simulink model "LqrTenzoWMotors"  (R2017a)
settings: Solver=ode23  StartTime=0.0  StopTime=15  RelTol=1e-3  EnableMultiTasking=on
values from neighbouring files (symbols this model uses):
  A0 = tenzo_min_nominale.a    [HTenzoV10.m]    (also in HTenzoV11.m; HTenzoV12.m; HTenzoV13.m; HTenzoV14.m)
  amplitudeNoise = 2    [HTenzoV10.m]    (also in HTenzoV11.m; HTenzoV12.m; HTenzoV13.m; HTenzoV14.m)
  amplitudePertIN = 0    [HTenzoV10.m]    (also in HTenzoV11.m; HTenzoV12.m; HTenzoV13.m; HTenzoV14.m)
  amplitudePertOut = 0    [HTenzoV10.m]    (also in HTenzoV11.m; HTenzoV12.m; HTenzoV13.m; HTenzoV14.m)
  Aoss = tenzo_min_nominale.a-L_3*tenzo_min_nominale.c    [HTenzoV10.m]    (also in HTenzoV11.m; HTenzoV12.m = tenzo_min_nominale.a-V*tenzo_min_nominale.c; HTenzoV13.m = tenzo_min_nominale.a-V*tenzo_min_nominale.c; HTenzoV14.m = tenzo_min_nominale.a-V*tenzo_min_nominale.c)
  B0 = tenzo_min_nominale.b    [HTenzoV10.m]    (also in HTenzoV11.m; HTenzoV12.m; HTenzoV13.m; HTenzoV14.m)
  Bossw = [tenzo_min_nominale.b-L_3*D L_3]    [HTenzoV10.m]    (also in HTenzoV11.m; HTenzoV12.m = [tenzo_min_nominale.b-V*D V]; HTenzoV13.m = [tenzo_min_nominale.b-V*D V]; HTenzoV14.m = [tenzo_min_nominale.b-V*D V])
  C0 = tenzo_min_nominale.c    [HTenzoV10.m]    (also in HTenzoV11.m; HTenzoV12.m; HTenzoV13.m; HTenzoV14.m)
  Coss = eye(size(Aoss,1))    [HTenzoV10.m]    (also in HTenzoV11.m; HTenzoV12.m; HTenzoV13.m; HTenzoV14.m)
  cstPertIn = 0    [HTenzoV10.m]    (also in HTenzoV11.m; HTenzoV12.m; HTenzoV13.m; HTenzoV14.m)
  cstPertOut = 0    [HTenzoV10.m]    (also in HTenzoV11.m; HTenzoV12.m; HTenzoV13.m; HTenzoV14.m)
  D0 = tenzo_min_nominale.d    [HTenzoV10.m]    (also in HTenzoV11.m; HTenzoV12.m; HTenzoV13.m; HTenzoV14.m)
  Doss = zeros(size(Aoss,1),poss)    [HTenzoV10.m]    (also in HTenzoV11.m; HTenzoV12.m; HTenzoV13.m; HTenzoV14.m)
  Kopt = Kopt_3    [HTenzoV10.m]    (also in HTenzoV11.m; HTenzoV12.m; HTenzoV13.m; HTenzoV14.m)
  omegaPertIN = 6    [HTenzoV10.m]    (also in HTenzoV11.m; HTenzoV12.m; HTenzoV13.m; HTenzoV14.m)
  omegaPertOut = 0.1    [HTenzoV10.m]    (also in HTenzoV11.m; HTenzoV12.m; HTenzoV13.m; HTenzoV14.m)
undefined symbols (not defined in the file or in its folder): sigbuilder_block
settings Model: SimulationMode=accelerator  Creator=danilo  LastModifiedBy=userk
settings DataIOCC: LimitDataPoints=on  SaveFormat=Array
settings OptimizationCC: ExpressionDepthLimit=2147483647  LifeSpan=inf
settings DebuggingCC: UnderspecifiedInitializationDetection=Classic  MergeDetectMultiDrivingBlocksExec=none  SolverPrmCheckMsg=warning  FcnCallInpInsideContextMsg=warning  AllowSymbolicDim=off  StateNameClashWarn=warning  SFUnexpectedBacktrackingDiag=warning  SFNoUnconditionalDefaultTransitionDiag=warning  SFExecutionAtInitializationDiag=none
settings HardwareCC: ProdBitPerPointer=32  ProdBitPerSizeT=32  ProdBitPerPtrDiffT=32  ProdLargestAtomicFloat=None  ProdIntDivRoundTo=Undefined  ProdEndianess=Unspecified  ProdWordSize=32  ProdHWDeviceType=32-bit Generic
settings ModelReferenceCC: PropagateSignalLabelsOutOfModel=off
settings GRTTargetCC: TargetLangStandard=C89/C90 (ANSI)  GeneratePreprocessorConditionals=Disable all  CombineOutputUpdateFcns=off  GRTInterface=on
settings ConfigComp: CovMetricSettings=dw  CovHtmlReporting=on  CovSaveCumulativeToWorkspaceVar=on  CovSaveSingleToWorkspaceVar=on  CovExternalEMLEnable=off

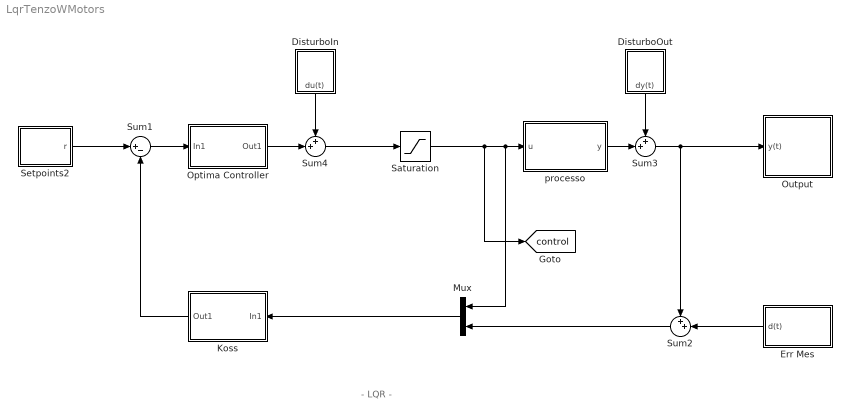
== system LqrTenzoWMotors ==
  note: - LQR -
  DisturboIn : Subsystem
  DisturboOut : Subsystem
  Err Mes : Subsystem
  Koss : Subsystem
  Mux : Mux  Inputs=2
  Optima Controller : Subsystem
  Output : Subsystem
  Saturation : Saturate  UpperLimit=36000000  LowerLimit=-36000000
  Setpoints2 : Subsystem
  Sum1 : Sum  Inputs=|+-
  Sum2 : Sum  Inputs=++|
  Sum3 : Sum  Inputs=++|
  Sum4 : Sum  Inputs=++|
  processo : Subsystem
  tag scope: control=global
  wires:
  Setpoints2/1(r) -> Sum1/1
  Err Mes/1("  d(t)") -> Sum2/2
  Sum2/1 -> Mux/2
  processo/1(y) -> Sum3/2
  Sum3/1 -> Sum2/1, Output/1(y(t))
  DisturboOut/1("dy(t) ") -> Sum3/1
  Sum1/1 -> Optima Controller/1(In1)
  Optima Controller/1(Out1) -> Sum4/2
  Mux/1 -> Koss/1(In1)
  Koss/1(Out1) -> Sum1/2
  DisturboIn/1(du(t)) -> Sum4/1
  Sum4/1 -> Saturation/1
  Saturation/1 -> [control], Mux/1, processo/1(u)

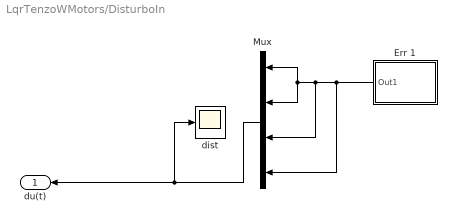
== system LqrTenzoWMotors/DisturboIn ==
  Err 1 : Subsystem
  Mux : Mux  Inputs=[1 1 1 1]
  dist : Scope
  du(t) : Outport
  wires:
  Mux/1 -> dist/1, du(t)/1
  Err 1/1(Out1) -> Mux/4, Mux/3, Mux/2, Mux/1

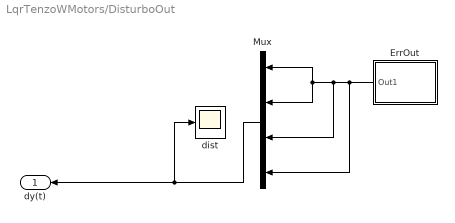
== system LqrTenzoWMotors/DisturboOut ==
  ErrOut : Subsystem
  Mux : Mux  Inputs=[1 1 1 1]
  dist : Scope
  "dy(t) " : Outport
  wires:
  ErrOut/1(Out1) -> Mux/4, Mux/3, Mux/2, Mux/1
  Mux/1 -> "dy(t) "/1, dist/1

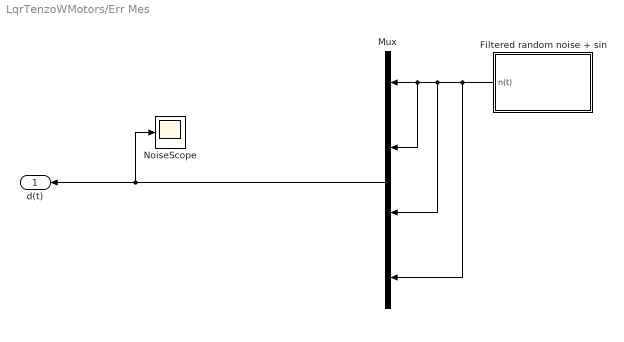
== system LqrTenzoWMotors/Err Mes ==
  Filtered random noise + sin : Subsystem
  Mux : Mux  Inputs=[1 1 1 1]
  NoiseScope : Scope
  "  d(t)" : Outport
  wires:
  Mux/1 -> NoiseScope/1, "  d(t)"/1
  Filtered random noise + sin/1(n(t)) -> Mux/4, Mux/3, Mux/2, Mux/1

== system LqrTenzoWMotors/Koss ==
  In1 : Inport
  "abc " : StateSpace  A=Aoss  B=Bossw  C=Coss  D=Doss  X0=0
  Out1 : Outport
  wires:
  In1/1 -> "abc "/1
  "abc "/1 -> Out1/1

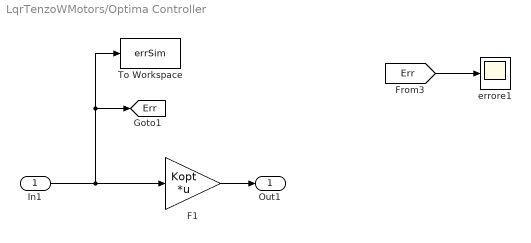
== system LqrTenzoWMotors/Optima Controller ==
  In1 : Inport
  F1 : Gain  Gain=Kopt  Multiplication=Matrix(K*u) (u vector)
  To Workspace : ToWorkspace  VariableName=errSim  SaveFormat=Structure  SampleTime=-1
  errore1 : Scope
  Out1 : Outport
  tag scope: Err=global
  wires:
  In1/1 -> F1/1, To Workspace/1, [Err]
  F1/1 -> Out1/1
  [Err] -> errore1/1

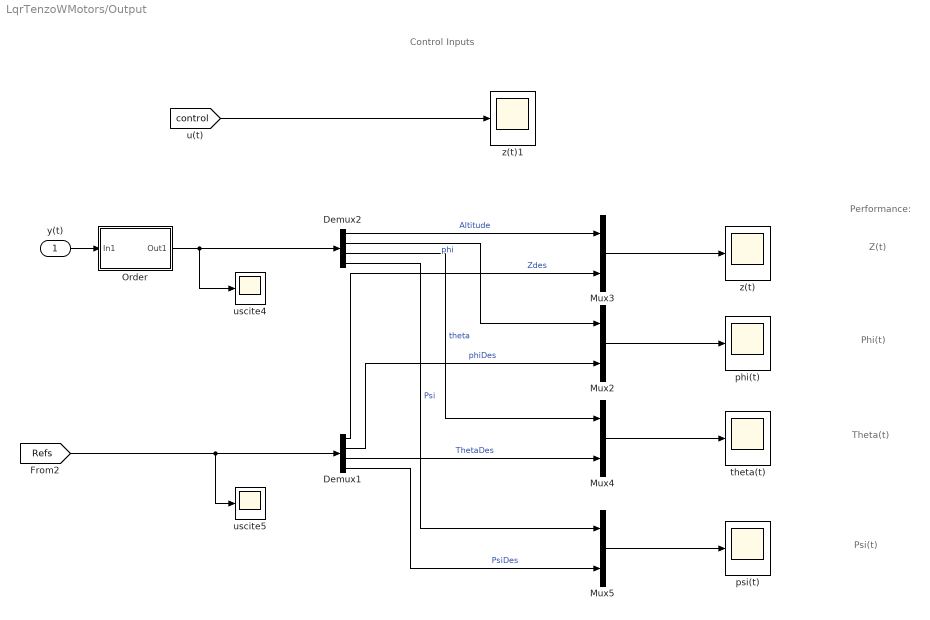
== system LqrTenzoWMotors/Output ==
  note: Psi(t)
  note: Theta(t)
  note: Phi(t)
  note: Performance:
  note: Z(t)
  note: Control Inputs
  y(t) : Inport
  Demux1 : Demux
  Demux2 : Demux
  Mux{2..5} (4 alike) : Mux  Inputs=2
  "Order " : Subsystem
  phi(t) : Scope
  psi(t) : Scope
  theta(t) : Scope
  uscite4 : Scope
  uscite5 : Scope
  z(t) : Scope
  z(t)1 : Scope
  wires:
  [Refs] -> Demux1/1, uscite5/1
  Demux1/1 -> Mux3/2  "Zdes"
  Mux2/1 -> phi(t)/1
  Demux2/2 -> Mux2/1  "phi"
  Mux3/1 -> z(t)/1
  Demux2/1 -> Mux3/1  "Altitude"
  Mux4/1 -> theta(t)/1
  Demux2/3 -> Mux4/1  "theta"
  Mux5/1 -> psi(t)/1
  Demux2/4 -> Mux5/1  "Psi"
  Demux1/2 -> Mux2/2  "phiDes"
  Demux1/3 -> Mux4/2  "ThetaDes"
  Demux1/4 -> Mux5/2  "PsiDes"
  "Order "/1(Out1) -> Demux2/1, uscite4/1
  y(t)/1 -> "Order "/1(In1)
  [control] -> z(t)1/1

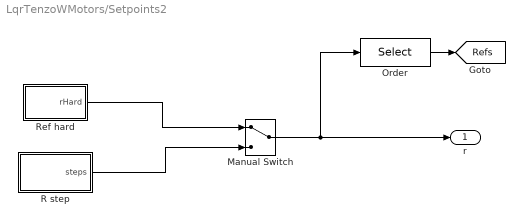
== system LqrTenzoWMotors/Setpoints2 ==
  Manual Switch : ManualSwitch
  Order : Selector  InputPortWidth=8  IndexOptions=Index vector (dialog)  Indices=[1,3,4,5]  OutputSizes=1
  R step : Subsystem
  "Ref hard " : Subsystem
  r : Outport
  tag scope: Refs=global
  wires:
  "Ref hard "/1(rHard) -> Manual Switch/1
  R step/1("steps ") -> Manual Switch/2
  Manual Switch/1 -> Order/1, r/1
  Order/1 -> [Refs]

== system LqrTenzoWMotors/processo ==
  u : Inport
  Processo1 : StateSpace  A=A0  B=B0  C=C0  D=D0  X0=0
  "u(t) " : Scope
  y : Outport
  wires:
  u/1 -> "u(t) "/1, Processo1/1
  Processo1/1 -> y/1

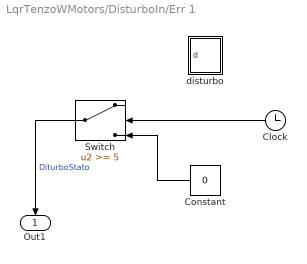
== system LqrTenzoWMotors/DisturboIn/Err 1 ==
  Clock : Clock
  Constant : Constant  Value=0
  Switch : Switch  Threshold=5
  disturbo : Subsystem
  Out1 : Outport
  wires:
  Constant/1 -> Switch/3
  Switch/1 -> Out1/1  "DiturboStato"
  Clock/1 -> Switch/2

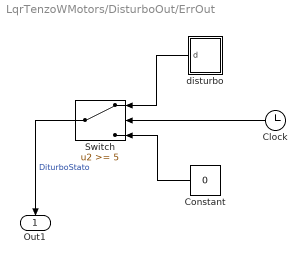
== system LqrTenzoWMotors/DisturboOut/ErrOut ==
  Clock : Clock
  Constant : Constant  Value=0
  Switch : Switch  Threshold=5
  disturbo : Subsystem
  Out1 : Outport
  wires:
  Clock/1 -> Switch/2
  Switch/1 -> Out1/1  "DiturboStato"
  disturbo/1(d) -> Switch/1
  Constant/1 -> Switch/3

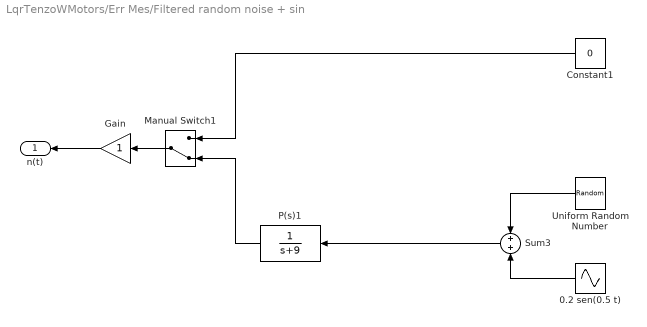
== system LqrTenzoWMotors/Err Mes/Filtered random noise + sin ==
  0.2 sen(0.5 t) : Sin  Amplitude=amplitudeNoise  Frequency=65  Phase=1  SampleTime=0
  Constant1 : Constant  Value=0
  Gain : Gain
  Manual Switch1 : ManualSwitch  CurrentSetting=0
  P(s)1 : TransferFcn  Numerator=1  Denominator=[1 9]
  Sum3 : Sum
  Uniform Random Number : UniformRandomNumber  Minimum=-10  Maximum=10  SampleTime=0.1
  n(t) : Outport
  wires:
  Uniform Random Number/1 -> Sum3/1
  Constant1/1 -> Manual Switch1/1
  Sum3/1 -> P(s)1/1
  Gain/1 -> n(t)/1
  P(s)1/1 -> Manual Switch1/2
  Manual Switch1/1 -> Gain/1
  0.2 sen(0.5 t)/1 -> Sum3/2

== system LqrTenzoWMotors/Output/Order  ==
  In1 : Inport
  Demux3 : Demux
  Mux1 : Mux
  Out1 : Outport
  wires:
  Demux3/2 -> Mux1/3
  Demux3/1 -> Mux1/2
  In1/1 -> Demux3/1
  Mux1/1 -> Out1/1
  Demux3/4 -> Mux1/1
  Demux3/3 -> Mux1/4

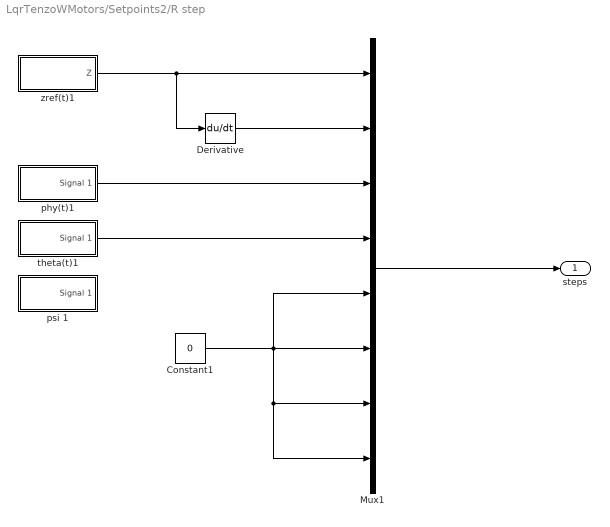
== system LqrTenzoWMotors/Setpoints2/R step ==
  Constant1 : Constant  Value=0
  Derivative : Derivative
  Mux1 : Mux  Inputs=[1 1 1 1 1 1 1 1]
  phy(t)1 : Subsystem  Tag=STV Subsys  LoadFcn=sigbuilder_block('load');  StartFcn=sigbuilder_block('start');  StopFcn=sigbuilder_block('stop');  ClipboardFcn=sigbuilder_block('clipboard');  mask(Sigbuilder block){tuvar=[0:10]}
      mask help: Simulink:masks:SigbuilderBlock_MD
      mask init:
      | if ~strcmp(get_param(bdroot(gcbh),'SimulationStatus'),'stopped') tuvar = sigbuilder_block('maskInit'); end
      settings: CopyFcn=sigbuilder_block('copy');  DeleteFcn=sigbuilder_block('delete');  ModelCloseFcn=sigbuilder_block('modelClose');  PreSaveFcn=sigbuilder_block('preSave');  PauseFcn=sigbuilder_block('pause');  ContinueFcn=sigbuilder_block('continue');  NameChangeFcn=sigbuilder_block('namechange');  OpenFcn=sigbuilder_block('open',[330 24 573 467.25 ]);  CloseFcn=sigbuilder_block('close');
      mask Display: plot(0, 0, 100, 100,[2, 2, 32, 32, 2], [68, 8, 8, 68, 68],[32, 2], [38, 38], [32, 19, 2],[53, 60, 44], [32, 17, 17, 2],[16, 16, 31, 31]);txt = getActiveGroup(gcbh);text(2, 100, txt,'verticalAlignment', 'top');
  psi 1 : Subsystem  Tag=STV Subsys  LoadFcn=sigbuilder_block('load');  StartFcn=sigbuilder_block('start');  StopFcn=sigbuilder_block('stop');  ClipboardFcn=sigbuilder_block('clipboard');  mask(Sigbuilder block){tuvar=[0:10]}
      mask help: Simulink:masks:SigbuilderBlock_MD
      mask init:
      | if ~strcmp(get_param(bdroot(gcbh),'SimulationStatus'),'stopped') tuvar = sigbuilder_block('maskInit'); end
      settings: CopyFcn=sigbuilder_block('copy');  DeleteFcn=sigbuilder_block('delete');  ModelCloseFcn=sigbuilder_block('modelClose');  PreSaveFcn=sigbuilder_block('preSave');  PauseFcn=sigbuilder_block('pause');  ContinueFcn=sigbuilder_block('continue');  NameChangeFcn=sigbuilder_block('namechange');  OpenFcn=sigbuilder_block('open',[326.25 -0.75 580.5 489.75 ]);  CloseFcn=sigbuilder_block('close');
      mask Display: plot(0, 0, 100, 100,[2, 2, 32, 32, 2], [68, 8, 8, 68, 68],[32, 2], [38, 38], [32, 19, 2],[53, 60, 44], [32, 17, 17, 2],[16, 16, 31, 31]);txt = getActiveGroup(gcbh);text(2, 100, txt,'verticalAlignment', 'top');
  theta(t)1 : Subsystem  Tag=STV Subsys  LoadFcn=sigbuilder_block('load');  StartFcn=sigbuilder_block('start');  StopFcn=sigbuilder_block('stop');  ClipboardFcn=sigbuilder_block('clipboard');  mask(Sigbuilder block){tuvar=[0:10]}
      mask help: Simulink:masks:SigbuilderBlock_MD
      mask init:
      | if ~strcmp(get_param(bdroot(gcbh),'SimulationStatus'),'stopped') tuvar = sigbuilder_block('maskInit'); end
      settings: CopyFcn=sigbuilder_block('copy');  DeleteFcn=sigbuilder_block('delete');  ModelCloseFcn=sigbuilder_block('modelClose');  PreSaveFcn=sigbuilder_block('preSave');  PauseFcn=sigbuilder_block('pause');  ContinueFcn=sigbuilder_block('continue');  NameChangeFcn=sigbuilder_block('namechange');  OpenFcn=sigbuilder_block('open',[333.75 27.75 565.5 444.75 ]);  CloseFcn=sigbuilder_block('close');
      mask Display: plot(0, 0, 100, 100,[2, 2, 32, 32, 2], [68, 8, 8, 68, 68],[32, 2], [38, 38], [32, 19, 2],[53, 60, 44], [32, 17, 17, 2],[16, 16, 31, 31]);txt = getActiveGroup(gcbh);text(2, 100, txt,'verticalAlignment', 'top');
  zref(t)1 : Subsystem  Tag=STV Subsys  LoadFcn=sigbuilder_block('load');  StartFcn=sigbuilder_block('start');  StopFcn=sigbuilder_block('stop');  ClipboardFcn=sigbuilder_block('clipboard');  mask(Sigbuilder block){tuvar=[0:10]}
      mask help: Simulink:masks:SigbuilderBlock_MD
      mask init:
      | if ~strcmp(get_param(bdroot(gcbh),'SimulationStatus'),'stopped') tuvar = sigbuilder_block('maskInit'); end
      settings: CopyFcn=sigbuilder_block('copy');  DeleteFcn=sigbuilder_block('delete');  ModelCloseFcn=sigbuilder_block('modelClose');  PreSaveFcn=sigbuilder_block('preSave');  PauseFcn=sigbuilder_block('pause');  ContinueFcn=sigbuilder_block('continue');  NameChangeFcn=sigbuilder_block('namechange');  OpenFcn=sigbuilder_block('open',[337.5 52.5 558 422.25 ]);  CloseFcn=sigbuilder_block('close');
      mask Display: plot(0, 0, 100, 100,[2, 2, 32, 32, 2], [68, 8, 8, 68, 68],[32, 2], [38, 38], [32, 19, 2],[53, 60, 44], [32, 17, 17, 2],[16, 16, 31, 31]);txt = getActiveGroup(gcbh);text(2, 100, txt,'verticalAlignment', 'top');
  "steps " : Outport
  wires:
  Constant1/1 -> Mux1/5, Mux1/8, Mux1/7, Mux1/6
  Mux1/1 -> "steps "/1
  theta(t)1/1(Signal 1) -> Mux1/4
  phy(t)1/1(Signal 1) -> Mux1/3
  zref(t)1/1(Z) -> Derivative/1, Mux1/1
  Derivative/1 -> Mux1/2

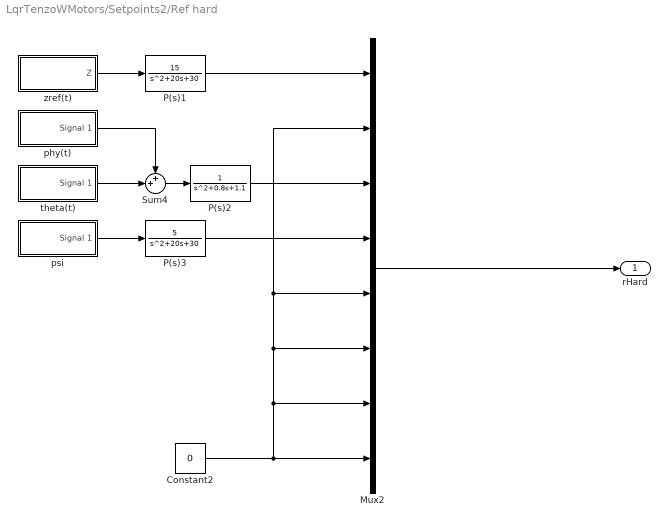
== system LqrTenzoWMotors/Setpoints2/Ref hard  ==
  Constant2 : Constant  Value=0
  Mux2 : Mux  Inputs=[1 1 1 1 1 1 1 1]
  P(s)1 : TransferFcn  Numerator=15  Denominator=[1 20 30]
  P(s)2 : TransferFcn  Numerator=1  Denominator=[1 0.8 1.1]
  P(s)3 : TransferFcn  Numerator=5  Denominator=[1 20 30]
  Sum4 : Sum  Inputs=++|
  phy(t) : Subsystem  Tag=STV Subsys  LoadFcn=sigbuilder_block('load');  StartFcn=sigbuilder_block('start');  StopFcn=sigbuilder_block('stop');  ClipboardFcn=sigbuilder_block('clipboard');  mask(Sigbuilder block){tuvar=[0:10]}
      mask help: Simulink:masks:SigbuilderBlock_MD
      mask init:
      | if ~strcmp(get_param(bdroot(gcbh),'SimulationStatus'),'stopped') tuvar = sigbuilder_block('maskInit'); end
      settings: CopyFcn=sigbuilder_block('copy');  DeleteFcn=sigbuilder_block('delete');  ModelCloseFcn=sigbuilder_block('modelClose');  PreSaveFcn=sigbuilder_block('preSave');  PauseFcn=sigbuilder_block('pause');  ContinueFcn=sigbuilder_block('continue');  NameChangeFcn=sigbuilder_block('namechange');  OpenFcn=sigbuilder_block('open',[333.75 48.75 565.5 444.75 ]);  CloseFcn=sigbuilder_block('close');
      mask Display: plot(0, 0, 100, 100,[2, 2, 32, 32, 2], [68, 8, 8, 68, 68],[32, 2], [38, 38], [32, 19, 2],[53, 60, 44], [32, 17, 17, 2],[16, 16, 31, 31]);txt = getActiveGroup(gcbh);text(2, 100, txt,'verticalAlignment', 'top');
  "psi " : Subsystem  Tag=STV Subsys  LoadFcn=sigbuilder_block('load');  StartFcn=sigbuilder_block('start');  StopFcn=sigbuilder_block('stop');  ClipboardFcn=sigbuilder_block('clipboard');  mask(Sigbuilder block){tuvar=[0:10]}
      mask help: Simulink:masks:SigbuilderBlock_MD
      mask init:
      | if ~strcmp(get_param(bdroot(gcbh),'SimulationStatus'),'stopped') tuvar = sigbuilder_block('maskInit'); end
      settings: CopyFcn=sigbuilder_block('copy');  DeleteFcn=sigbuilder_block('delete');  ModelCloseFcn=sigbuilder_block('modelClose');  PreSaveFcn=sigbuilder_block('preSave');  PauseFcn=sigbuilder_block('pause');  ContinueFcn=sigbuilder_block('continue');  NameChangeFcn=sigbuilder_block('namechange');  OpenFcn=sigbuilder_block('open',[330 24 573 467.25 ]);  CloseFcn=sigbuilder_block('close');
      mask Display: plot(0, 0, 100, 100,[2, 2, 32, 32, 2], [68, 8, 8, 68, 68],[32, 2], [38, 38], [32, 19, 2],[53, 60, 44], [32, 17, 17, 2],[16, 16, 31, 31]);txt = getActiveGroup(gcbh);text(2, 100, txt,'verticalAlignment', 'top');
  theta(t) : Subsystem  Tag=STV Subsys  LoadFcn=sigbuilder_block('load');  StartFcn=sigbuilder_block('start');  StopFcn=sigbuilder_block('stop');  ClipboardFcn=sigbuilder_block('clipboard');  mask(Sigbuilder block){tuvar=[0:10]}
      mask help: Simulink:masks:SigbuilderBlock_MD
      mask init:
      | if ~strcmp(get_param(bdroot(gcbh),'SimulationStatus'),'stopped') tuvar = sigbuilder_block('maskInit'); end
      settings: CopyFcn=sigbuilder_block('copy');  DeleteFcn=sigbuilder_block('delete');  ModelCloseFcn=sigbuilder_block('modelClose');  PreSaveFcn=sigbuilder_block('preSave');  PauseFcn=sigbuilder_block('pause');  ContinueFcn=sigbuilder_block('continue');  NameChangeFcn=sigbuilder_block('namechange');  OpenFcn=sigbuilder_block('open',[333.75 48.75 565.5 444.75 ]);  CloseFcn=sigbuilder_block('close');
      mask Display: plot(0, 0, 100, 100,[2, 2, 32, 32, 2], [68, 8, 8, 68, 68],[32, 2], [38, 38], [32, 19, 2],[53, 60, 44], [32, 17, 17, 2],[16, 16, 31, 31]);txt = getActiveGroup(gcbh);text(2, 100, txt,'verticalAlignment', 'top');
  zref(t) : Subsystem  Tag=STV Subsys  LoadFcn=sigbuilder_block('load');  StartFcn=sigbuilder_block('start');  StopFcn=sigbuilder_block('stop');  ClipboardFcn=sigbuilder_block('clipboard');  mask(Sigbuilder block){tuvar=[0:10]}
      mask help: Simulink:masks:SigbuilderBlock_MD
      mask init:
      | if ~strcmp(get_param(bdroot(gcbh),'SimulationStatus'),'stopped') tuvar = sigbuilder_block('maskInit'); end
      settings: CopyFcn=sigbuilder_block('copy');  DeleteFcn=sigbuilder_block('delete');  ModelCloseFcn=sigbuilder_block('modelClose');  PreSaveFcn=sigbuilder_block('preSave');  PauseFcn=sigbuilder_block('pause');  ContinueFcn=sigbuilder_block('continue');  NameChangeFcn=sigbuilder_block('namechange');  OpenFcn=sigbuilder_block('open',[341.25 77.25 550.5 399.75 ]);  CloseFcn=sigbuilder_block('close');
      mask Display: plot(0, 0, 100, 100,[2, 2, 32, 32, 2], [68, 8, 8, 68, 68],[32, 2], [38, 38], [32, 19, 2],[53, 60, 44], [32, 17, 17, 2],[16, 16, 31, 31]);txt = getActiveGroup(gcbh);text(2, 100, txt,'verticalAlignment', 'top');
  rHard : Outport
  wires:
  "psi "/1(Signal 1) -> P(s)3/1
  Sum4/1 -> P(s)2/1
  P(s)2/1 -> Mux2/3
  zref(t)/1(Z) -> P(s)1/1
  Mux2/1 -> rHard/1
  Constant2/1 -> Mux2/8, Mux2/7, Mux2/6, Mux2/2, Mux2/5
  theta(t)/1(Signal 1) -> Sum4/2
  P(s)1/1 -> Mux2/1
  phy(t)/1(Signal 1) -> Sum4/1
  P(s)3/1 -> Mux2/4

== system LqrTenzoWMotors/DisturboIn/Err 1/disturbo ==
  Constant : Constant  Value=cstPertIn
  Sine Wave : Sin  Amplitude=amplitudePertIN  Frequency=omegaPertIN  SampleTime=0
  Sum2 : Sum  Inputs=|++
  d : Outport
  wires:
  Sum2/1 -> d/1
  Constant/1 -> Sum2/1
  Sine Wave/1 -> Sum2/2

== system LqrTenzoWMotors/DisturboOut/ErrOut/disturbo ==
  Constant : Constant  Value=cstPertOut
  SinOut : Sin  Amplitude=amplitudePertOut  Frequency=omegaPertOut  SampleTime=0
  Sum2 : Sum  Inputs=|++
  d : Outport
  wires:
  SinOut/1 -> Sum2/2
  Constant/1 -> Sum2/1
  Sum2/1 -> d/1

== system LqrTenzoWMotors/Setpoints2/R step/phy(t)1 ==
  Demux : Demux  Tag=STV Demux  Outputs=1
  FromWs : FromWorkspace  Tag=STV FromWs  VariableName=tuvar  SampleTime=0
      SigBuilderData=|
      | common.afterFinalStr = 'Extrapolate'
      | common.sampleTime = 0
      | dataSet.timeRange = [0 10]
      | dataSet.name = 'Group 1'
      | sbobj.Groups.Name = 'Group 1'
      | sbobj.Groups.Signals.Name = 'Signal 1'
      | sbobj.Groups.Signals.XData = [0 0.98 1 10]
      | sbobj.Groups.Signals.YData = [0 0 50 50]
  Signal 1 : Outport  Tag=STV Outport
  wires:
  Demux/1 -> Signal 1/1
  FromWs/1 -> Demux/1

== system LqrTenzoWMotors/Setpoints2/R step/psi 1 ==
  Demux : Demux  Tag=STV Demux  Outputs=1
  FromWs : FromWorkspace  Tag=STV FromWs  VariableName=tuvar  SampleTime=0
      SigBuilderData=|
      | common.afterFinalStr = 'Extrapolate'
      | common.sampleTime = 0
      | dataSet.timeRange = [0 15]
      | dataSet.name = 'Group 1'
      | sbobj.Groups.Name = 'Group 1'
      | sbobj.Groups.Signals.Name = 'Signal 1'
      | sbobj.Groups.Signals.XData = [0 2.1 2.1 15]
      | sbobj.Groups.Signals.YData = [0 0 10 10]
      | sbobj.Groups.TimeRange = [0 15]
  Signal 1 : Outport  Tag=STV Outport
  wires:
  Demux/1 -> Signal 1/1
  FromWs/1 -> Demux/1

== system LqrTenzoWMotors/Setpoints2/R step/theta(t)1 ==
  Demux : Demux  Tag=STV Demux  Outputs=1
  FromWs : FromWorkspace  Tag=STV FromWs  VariableName=tuvar  SampleTime=0
      SigBuilderData=|
      | common.afterFinalStr = 'Extrapolate'
      | common.sampleTime = 0
      | dataSet.timeRange = [0 10]
      | dataSet.name = 'Group 1'
      | sbobj.Groups.Name = 'Group 1'
      | sbobj.Groups.Signals.Name = 'Signal 1'
      | sbobj.Groups.Signals.XData = [0 1 1 10]
      | sbobj.Groups.Signals.YData = [0 0 10 10]
  Signal 1 : Outport  Tag=STV Outport
  wires:
  Demux/1 -> Signal 1/1
  FromWs/1 -> Demux/1

== system LqrTenzoWMotors/Setpoints2/R step/zref(t)1 ==
  Demux : Demux  Tag=STV Demux  Outputs=1
  FromWs : FromWorkspace  Tag=STV FromWs  VariableName=tuvar  SampleTime=0
      SigBuilderData=|
      | common.afterFinalStr = 'Extrapolate'
      | common.sampleTime = 0
      | dataSet.timeRange = [0 10]
      | dataSet.name = 'Group 1'
      | sbobj.Groups.Name = 'Group 1'
      | sbobj.Groups.Signals.Name = 'Z'
      | sbobj.Groups.Signals.XData = [0 1 1 6.82 10]
      | sbobj.Groups.Signals.YData = [0 0 10 10 10]
  Z : Outport  Tag=STV Outport
  wires:
  FromWs/1 -> Demux/1
  Demux/1 -> Z/1

== system LqrTenzoWMotors/Setpoints2/Ref hard /phy(t) ==
  Demux : Demux  Tag=STV Demux  Outputs=1
  FromWs : FromWorkspace  Tag=STV FromWs  VariableName=tuvar  SampleTime=0
      SigBuilderData=|
      | common.afterFinalStr = 'Extrapolate'
      | common.sampleTime = 0
      | dataSet.timeRange = [0 10]
      | dataSet.name = 'Group 1'
      | sbobj.Groups.Name = 'Group 1'
      | sbobj.Groups.Signals.Name = 'Signal 1'
      | sbobj.Groups.Signals.XData = [0 0.98 2 7 7.14 10]
      | sbobj.Groups.Signals.YData = [0 0 50 50 0 0]
  Signal 1 : Outport  Tag=STV Outport
  wires:
  Demux/1 -> Signal 1/1
  FromWs/1 -> Demux/1

== system LqrTenzoWMotors/Setpoints2/Ref hard /psi  ==
  Demux : Demux  Tag=STV Demux  Outputs=1
  FromWs : FromWorkspace  Tag=STV FromWs  VariableName=tuvar  SampleTime=0
      SigBuilderData=|
      | common.afterFinalStr = 'Extrapolate'
      | common.sampleTime = 0
      | dataSet.timeRange = [0 15]
      | dataSet.name = 'Group 1'
      | sbobj.Groups.Name = 'Group 1'
      | sbobj.Groups.Signals.Name = 'Signal 1'
      | sbobj.Groups.Signals.XData = [0 2.1 2.6 6.82 10 15]
      | sbobj.Groups.Signals.YData = [0 0 150 150 0 0]
      | sbobj.Groups.TimeRange = [0 15]
  Signal 1 : Outport  Tag=STV Outport
  wires:
  Demux/1 -> Signal 1/1
  FromWs/1 -> Demux/1

== system LqrTenzoWMotors/Setpoints2/Ref hard /theta(t) ==
  Demux : Demux  Tag=STV Demux  Outputs=1
  FromWs : FromWorkspace  Tag=STV FromWs  VariableName=tuvar  SampleTime=0
      SigBuilderData=|
      | common.afterFinalStr = 'Extrapolate'
      | common.sampleTime = 0
      | dataSet.timeRange = [0 10]
      | dataSet.name = 'Group 1'
      | sbobj.Groups.Name = 'Group 1'
      | sbobj.Groups.Signals.Name = 'Signal 1'
      | sbobj.Groups.Signals.XData = [0 1 2.06 4.06 4.14 10]
      | sbobj.Groups.Signals.YData = [0 0 10 10 0 0]
  Signal 1 : Outport  Tag=STV Outport
  wires:
  Demux/1 -> Signal 1/1
  FromWs/1 -> Demux/1

== system LqrTenzoWMotors/Setpoints2/Ref hard /zref(t) ==
  Demux : Demux  Tag=STV Demux  Outputs=1
  FromWs : FromWorkspace  Tag=STV FromWs  VariableName=tuvar  SampleTime=0
      SigBuilderData=|
      | common.afterFinalStr = 'Extrapolate'
      | common.sampleTime = 0
      | dataSet.timeRange = [0 10]
      | dataSet.name = 'Group 1'
      | sbobj.Groups.Name = 'Group 1'
      | sbobj.Groups.Signals.Name = 'Z'
      | sbobj.Groups.Signals.XData = [0 1 2.06 6.82 6.82 10]
      | sbobj.Groups.Signals.YData = [0 0 10 10 0 0]
  Z : Outport  Tag=STV Outport
  wires:
  FromWs/1 -> Demux/1
  Demux/1 -> Z/1
